simulink model "miniProject3"  (Simulink 7.7)
settings: Solver=ode45  StartTime=0.0  StopTime=1000  RelTol=1e-3
settings Model: Creator=jiannianweng  LastModifiedBy=jiannianweng
settings DebuggingCC: SolverPrmCheckMsg=none

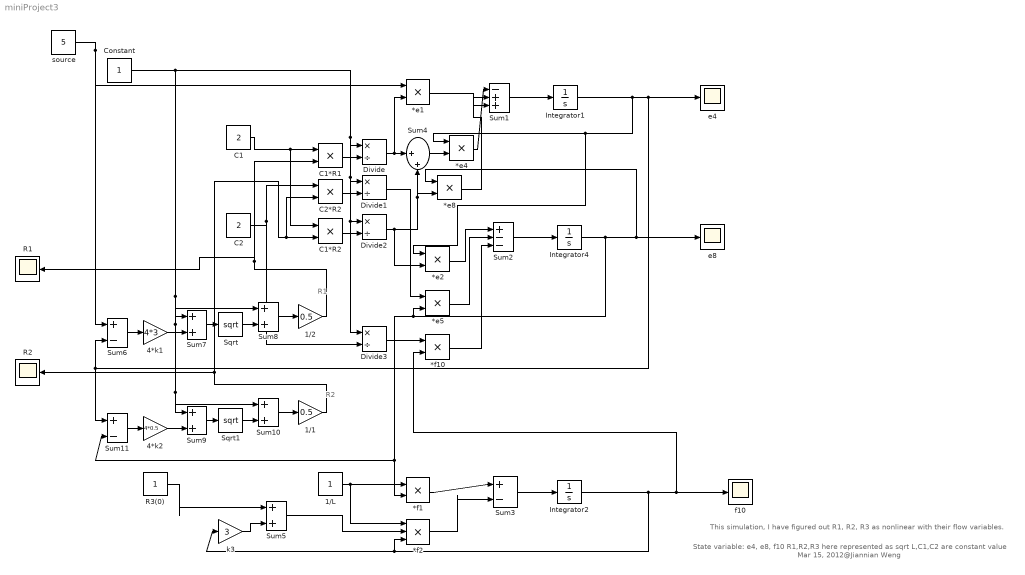
== system miniProject3 ==
  note: State variable: e4, e8, f10
      | R1,R2,R3 here represented as sqrt
      | L,C1,C2 are constant value
      | Mar 15, 2012@Jiannian Weng
  note: This simulation, I have figured out R1, R2, R3 as nonlinear
      | with their flow variables.
  note: R1
  note: R2
  *e{1..2,4..5,8} (5 alike) : Product  RndMeth=Zero
  *f1 : Product  RndMeth=Zero
  *f10 : Product  RndMeth=Zero
  *f2 : Product  Inputs=3  RndMeth=Zero
  1/1 : Gain  Gain=0.5
  1/2 : Gain  Gain=0.5
  1/L : Constant
  4*k1 : Gain  Gain=4*3
  4*k2 : Gain  Gain=4*0.5
  C1 : Constant  Value=2
  C1*R1 : Product  RndMeth=Zero
  C1*R2 : Product  RndMeth=Zero
  C2 : Constant  Value=2
  C2*R2 : Product  RndMeth=Zero
  Constant : Constant
  Divide{,1..3} (4 alike) : Product  Inputs=*/
  Integrator1 : Integrator
  Integrator2 : Integrator
  Integrator4 : Integrator
  R1 : Scope
      settings: YMin=0.67614  YMax=0.676142  SaveName=ScopeData3
  R2 : Scope
      settings: YMin=0.67614  YMax=0.676142  SaveName=ScopeData4
  R3(0) : Constant
  Sqrt : Sqrt  OutputSignalType=real  SaturateOnIntegerOverflow=on
  Sqrt1 : Sqrt  OutputSignalType=real  SaturateOnIntegerOverflow=on
  Sum1 : Sum  Inputs=|-++
  Sum{4..5,7..10} (6 alike) : Sum  Inputs=|++
  Sum11 : Sum  Inputs=|+-
  Sum2 : Sum  Inputs=|+--
  Sum3 : Sum  Inputs=|+-
  Sum6 : Sum  Inputs=|+-
  e4 : Scope
      settings: YMin=0.67614  YMax=0.676142
  e8 : Scope
      settings: YMin=0.67614  YMax=0.676142
  f10 : Scope
      settings: YMin=0.67614  YMax=0.676142  SaveName=ScopeData2
  k3 : Gain  Gain=3
  source : Constant  Value=5
  wires:
  Sum3/1 -> Integrator2/1
  Integrator1/1 -> *e4/1, *e2/1, e4/1, Sum6/2, Sum11/1
  Integrator4/1 -> e8/1, *e8/1, *e5/2, *f1/2, Sum11/2
  Sum1/1 -> Integrator1/1
  Sum2/1 -> Integrator4/1
  C1/1 -> C1*R1/1, C1*R2/1
  1/2/1 -> C1*R1/2, R1/1
  C1*R1/1 -> Divide/2
  Constant/1 -> Divide/1, Divide1/1, Divide2/1, Divide3/1, Sum8/1, Sum7/1, Sum9/1, Sum10/1
  C2/1 -> C2*R2/1, Divide3/2
  C2*R2/1 -> Divide1/2
  C1*R2/1 -> Divide2/2
  Divide/1 -> Sum4/1, *e1/2
  Divide2/1 -> Sum4/2, *e8/2, *e2/2
  Sum4/1 -> *e4/2
  *e4/1 -> Sum1/1
  source/1 -> Sum6/1, *e1/1
  *e8/1 -> Sum1/2
  *e2/1 -> Sum2/1
  Divide1/1 -> *e5/1
  *e5/1 -> Sum2/2
  Integrator2/1 -> f10/1, *f10/2, *f2/3, k3/1
  Divide3/1 -> *f10/1
  *f10/1 -> Sum2/3
  1/L/1 -> *f1/1, *f2/1
  *f1/1 -> Sum3/1
  *f2/1 -> Sum3/2
  R3(0)/1 -> Sum5/1
  k3/1 -> Sum5/2
  Sum5/1 -> *f2/2
  Sum6/1 -> 4*k1/1
  4*k1/1 -> Sum7/2
  Sum7/1 -> Sqrt/1
  Sqrt/1 -> Sum8/2
  Sum8/1 -> 1/2/1
  4*k2/1 -> Sum9/2
  Sum9/1 -> Sqrt1/1
  Sqrt1/1 -> Sum10/2
  Sum10/1 -> 1/1/1
  1/1/1 -> C1*R2/2, C2*R2/2, R2/1
  Sum11/1 -> 4*k2/1
  *e1/1 -> Sum1/3
